simulink model "CruiseControl_withController"  (R2020a)
settings: Solver=VariableStepAuto  StartTime=0.0  StopTime=120  RelTol=1e-3
values from neighbouring files (symbols this model uses):
  Kd = 1.0    [Datadictionary_CruiseControl.sldd]
  Ki = 40.0    [Datadictionary_CruiseControl.sldd]
  Kp = 800.0    [Datadictionary_CruiseControl.sldd]
settings Model: DataDictionary=Datadictionary_CruiseControl.sldd  Creator=DELL  LastModifiedBy=DELL

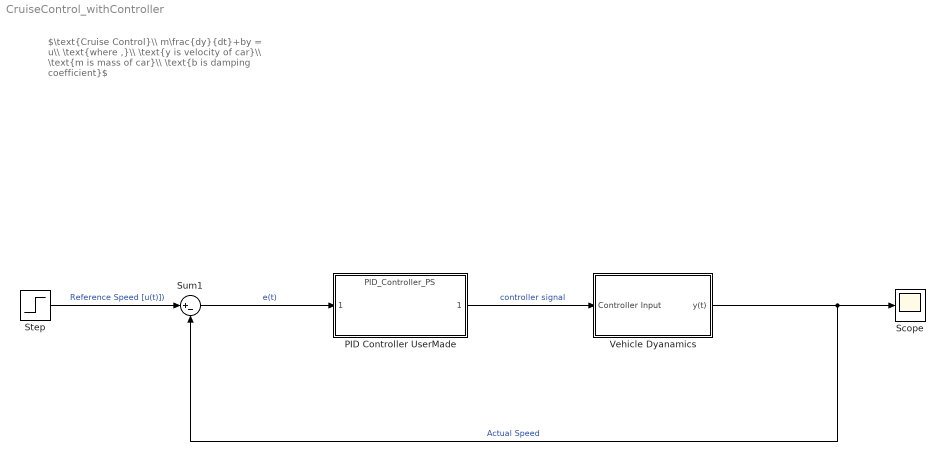
== system CruiseControl_withController ==
  note: $\text{Cruise Control}\\ m\frac{dy}{dt}+by = u\\ \text{where ,}\\ \text{y is velocity of car}\\ \text{m is mass of car}\\ \text{b is damping coefficient}$
  PID Controller UserMade : ModelReference  ModelNameDialog=PID_Controller_PS  ParameterArgumentNames=Kd,Ki,Kp  ParameterArgumentValues=Kd,Ki,Kp  UsingDefaultArgumentValue=0,0,0  SimulationMode=Normal  ModelReferenceVersion=1.19  Kd=1  Ki=44  Kp=335  SimulationMode=Normal
  Scope : Scope
  Step : Step  Time=0  After=u  SampleTime=0
  Sum1 : Sum  Inputs=|+-
  Vehicle Dyanamics : Subsystem  mask{m=1000, b=50}
      mask prompts: m "Inertia of Vehicle (m)"; b "Damping coefficient (b)"
      mask DialogControl DescGroupVar Prompt: Vehical
      mask DialogControl DescTextVar Prompt: Vehical dynamics parameters.
  wires:
  Vehicle Dyanamics/1(y(t)) -> Sum1/2, Scope/1  "Actual Speed"
  Sum1/1 -> PID Controller UserMade/1  "e(t)"
  PID Controller UserMade/1 -> Vehicle Dyanamics/1(Controller Input)  "controller signal"
  Step/1 -> Sum1/1  "Reference Speed [u(t)])"

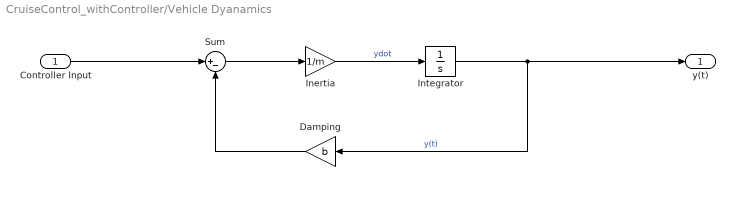
== system CruiseControl_withController/Vehicle Dyanamics ==
  Controller Input : Inport
  Damping : Gain  Gain=b
  Inertia : Gain  Gain=1/m
  Integrator : Integrator
  Sum : Sum  Inputs=|+-
  y(t) : Outport
  wires:
  Controller Input/1 -> Sum/1
  Inertia/1 -> Integrator/1  "ydot"
  Integrator/1 -> y(t)/1, Damping/1  "y(t)"
  Damping/1 -> Sum/2
  Sum/1 -> Inertia/1
